simulink model "P4p2_integral"  (R2015a)
settings: Solver=ode1  StartTime=0.0  StopTime=inf  FixedStep=0.002  RelTol=1e-3
PostLoadFcn:
  | qc_set_target_type(getConfigSet(bdroot, 'QUARC Default Target Configuration'));
values from neighbouring files (symbols this model uses):
  A_hat = [0 1 0 0 0 0; zeros(1, 6); 0 0 0 1 0 0;zeros(1, 6); 0 0 0 0 0 1; k_3 0 0 0 0 0]    [P4p2_init.m]    (also in P4p3_init.m; p4p2_integral_init.m)
  B_hat = [0 0 ;0 k_1; 0 0; k_2 0; 0 0; 0 0]    [P4p2_init.m]    (also in P4p3_init.m; p4p2_integral_init.m)
  C_hat = [[1 0 0 0 0 0];[0 0 1 0 0 0]; [0 0 0 0 1 0]]    [P4p2_init.m]    (also in P4p3_init.m = [[0 0 1 0 0 0]; [0 0 0 0 1 0]]; p4p2_integral_init.m)
  K = lqr(A_reg, B_reg, Q_reg, R_reg)    [P4p2_init.m]    (also in P4p3_init.m; p4p2_integral_init.m)
  L = place(A_hat', C_hat', poles)'    [P4p2_init.m]    (also in P4p3_init.m; p4p2_integral_init.m)
  P = inv(C_reg*inv(B_reg*K-A_reg)*B_reg)    [P4p2_init.m]    (also in P4p3_init.m = inv(C*inv(B*K_new-A)*B); p4p2_integral_init.m = inv(C*inv(B*K_new-A)*B))
undefined symbols (not defined in the file or in its folder): HIL, Joystick_gain_x, Joystick_gain_y, qc_get_step_size, V_ss
libraries: simulink_extras x6, quarc_library x4
settings Model: SimulationMode=external  CovSFcnEnable=off  ExtModeTrigDuration=1000000  Creator=Rchan  LastModifiedBy=aashil
settings SolverCC: PositivePriorityOrder=on
settings DataIOCC: SignalLoggingSaveFormat=ModelDataLogs
settings OptimizationCC: ExpressionDepthLimit=2147483647  InitFltsAndDblsToZero=on
settings DebuggingCC: SaveWithParameterizedLinksMsg=none  UnderspecifiedInitializationDetection=Classic  MergeDetectMultiDrivingBlocksExec=none  SolverPrmCheckMsg=warning  MultiTaskDSMMsg=warning  MultiTaskCondExecSysMsg=none  FcnCallInpInsideContextMsg=UseLocalSettings  StateNameClashWarn=warning
settings RTWCC: SystemTargetFile=quarc_win64.tlc  TemplateMakefile=quarc_default_tmf  Description=QUARC Win64 Target
settings STFCustomTargetCC: TargetLibSuffix=.lib  TargetPreCompLibLocation=C:\PROGRA~3\QUARC\lib\2014a\win64\release  GenerateSampleERTMain=off  ConcurrentExecutionCompliant=on  GeneratePreprocessorConditionals=Disable all  ERTCustomFileBanners=off  SupportNonInlinedSFcns=on  SupportVariableSizeSignals=off  MATLABClassNameForMDSCustomization=Simulink.SoftwareTarget.GRTCustomization  CPPClassGenCompliant=on  GRTInterface=on  SystemTargetFile=quarc_win64.tlc
settings GRTTargetCC: TargetPreCompLibLocation=C:\PROGRA~3\QUARC\lib\2014a\win64\release  ParMdlRefBuildCompliant=off  CompOptLevelCompliant=off  CombineOutputUpdateFcns=off  MatFileLogging=off  GRTInterface=on  ExtMode=on  ExtModeMexFile=quarc_comm

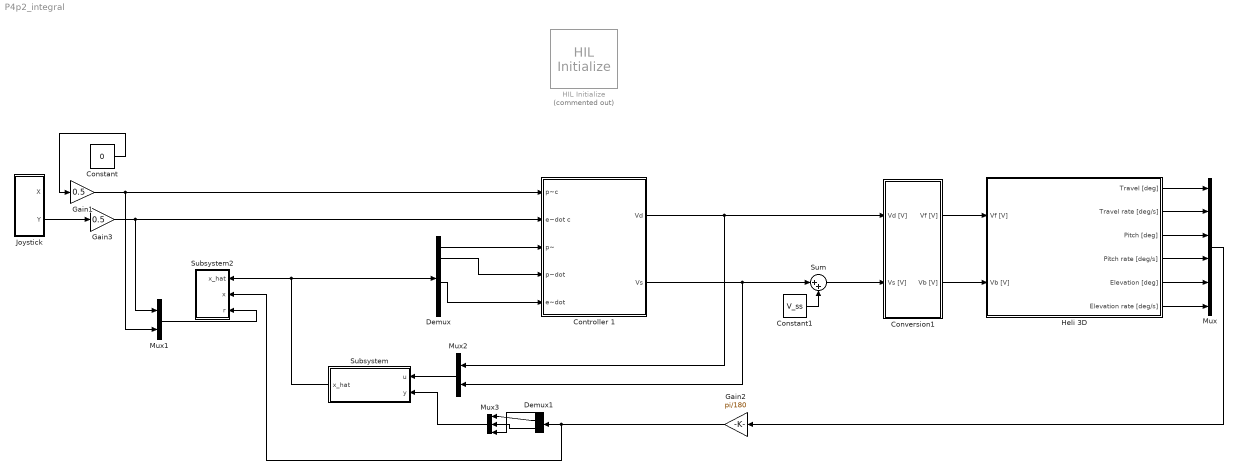
== system P4p2_integral ==
  Constant : Constant  Value=0
  Constant1 : Constant  Value=V_ss
  Controller 1 : Subsystem
  Conversion1 : Subsystem
  Demux : Demux  Outputs=6
  Demux1 : Demux  Outputs=6
  Gain1 : Gain  Gain=0.5
  Gain2 : Gain  Gain=pi/180
  Gain3 : Gain  Gain=0.5
  HIL Initialize : quarc_library/Data Acquisition/Generic/Configuration/HIL Initialize  Priority=-99  Commented=on  object_name=HIL-1  board_type=q8_usb  board_number=0  board_options=update_rate=normal;decimation=1  exclusive=off  active=off  hardware_clocks=[0:2]  clock_modes=[]  initial_clock_frequencies=[]  set_clock_params_at_start=off  set_clock_params_at_switch_in=off  set_clock_frequencies_at_start=off  set_clock_frequencies_at_switch_in=off  analog_input_channels=[0:7]  analog_input_maximums=10  analog_input_minimums=-10  set_analog_input_params_at_start=on  set_analog_input_params_at_switch_in=off  analog_output_channels=[0:7]  analog_output_maximums=10  analog_output_minimums=-10  initial_analog_outputs=[0]  final_analog_outputs=[0]  watchdog_analog_outputs=0  set_analog_output_params_at_start=on  set_analog_output_params_at_switch_in=off  set_analog_outputs_at_start=on  set_analog_outputs_at_switch_in=off  set_analog_outputs_at_terminate=on  set_analog_outputs_at_switch_out=off  set_analog_outputs_on_watchdog=off  digital_input_channels=[]  digital_output_channels=[]  digital_output_configuration=[]  initial_digital_outputs=[1]  final_digital_outputs=[1]  watchdog_digital_outputs=[1]  set_digital_output_params_at_start=off  set_digital_output_params_at_switch_in=off  set_digital_outputs_at_start=on  set_digital_outputs_at_switch_in=off  set_digital_outputs_at_terminate=on  set_digital_outputs_at_switch_out=off  set_digital_outputs_on_watchdog=off  encoder_channels=[0:7]  quadrature=[4]  encoder_filter_frequency=[]  initial_encoder_counts=[0]  set_encoder_params_at_start=on  set_encoder_params_at_switch_in=off  set_encoder_counts_at_start=on  set_encoder_counts_at_switch_in=off  pwm_channels=[0:7]  pwm_modes=0  pwm_frequency=99.532799999999995e6/4095  pwm_configuration=[0]  pwm_alignment=[0]  pwm_polarity=[1]  pwm_leading_deadband=[0]  pwm_trailing_deadband=[0]  initial_pwm_outputs=[0]  final_pwm_outputs=[0]  watchdog_pwm_outputs=[0]  set_pwm_params_at_start=on  set_pwm_params_at_switch_in=off  set_pwm_outputs_at_start=on  set_pwm_outputs_at_switch_in=off  set_pwm_outputs_at_terminate=on  set_pwm_outputs_at_switch_out=off  set_pwm_outputs_on_watchdog=off  other_output_channels=[]  initial_other_outputs=[]  final_other_outputs=[]  watchdog_other_outputs=[]  set_other_outputs_at_start=off  set_other_outputs_at_switch_in=off  set_other_outputs_at_terminate=off  set_other_outputs_at_switch_out=off  set_other_outputs_on_watchdog=off
  Heli 3D : Subsystem
  Joystick : Subsystem
  Mux : Mux  Inputs=6
  Mux1 : Mux  Inputs=2
  Mux2 : Mux  Inputs=2
  Mux3 : Mux  Inputs=3
  Subsystem : Subsystem
  Subsystem2 : Subsystem
  Sum : Sum  Inputs=|++
  wires:
  Conversion1/2(Vb [V]) -> Heli 3D/2(Vb [V])
  Conversion1/1(Vf [V]) -> Heli 3D/1(Vf [V])
  Heli 3D/1(Travel [deg]) -> Mux/1
  Heli 3D/2(Travel rate [deg/s]) -> Mux/2
  Heli 3D/3(Pitch [deg]) -> Mux/3
  Heli 3D/4(Pitch rate [deg/s]) -> Mux/4
  Heli 3D/5(Elevation [deg]) -> Mux/5
  Heli 3D/6(Elevation rate [deg/s]) -> Mux/6
  Mux/1 -> Gain2/1
  Joystick/2(Y) -> Gain3/1
  Gain3/1 -> Mux1/1, Controller 1/2(e~dot c)
  Constant/1 -> Gain1/1
  Mux1/1 -> Subsystem2/3(r)
  Gain1/1 -> Controller 1/1(p~c), Mux1/2
  Mux2/1 -> Subsystem/1(u)
  Subsystem/1(x_hat) -> Demux/1, Subsystem2/1(x_hat)
  Demux1/1 -> Mux3/3
  Demux1/3 -> Mux3/1
  Demux1/5 -> Mux3/2
  Mux3/1 -> Subsystem/2(y)
  Demux/1 -> Controller 1/3(p~)
  Demux/2 -> Controller 1/4(p~dot)
  Gain2/1 -> Subsystem2/2(x), Demux1/1
  Demux/4 -> Controller 1/5(e~dot)
  Controller 1/1("Vd ") -> Mux2/1, Conversion1/1(Vd [V])
  Constant1/1 -> Sum/2
  Sum/1 -> Conversion1/2(Vs [V])
  Controller 1/2(Vs) -> Sum/1, Mux2/2

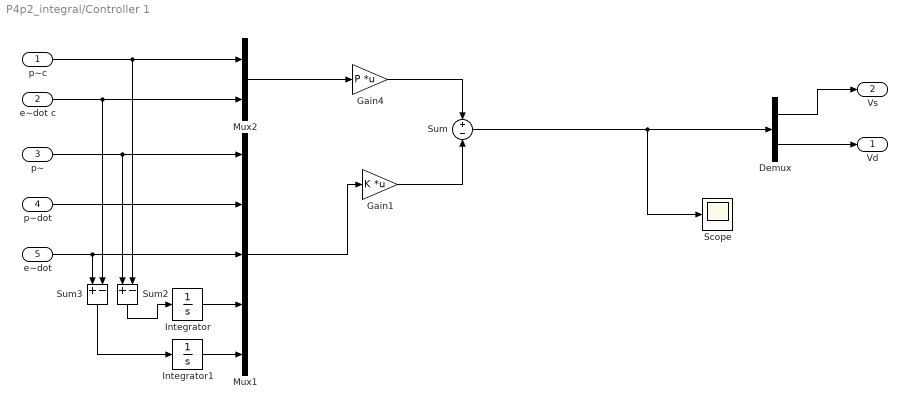
== system P4p2_integral/Controller 1 ==
  p~c : Inport
  e~dot c : Inport  Port=2
  p~ : Inport  Port=3
  p~dot : Inport  Port=4
  e~dot : Inport  Port=5
  Demux : Demux  Outputs=2
  Gain1 : Gain  Gain=K  Multiplication=Matrix(K*u)
  Gain4 : Gain  Gain=P  Multiplication=Matrix(K*u)
  Integrator : Integrator
  Integrator1 : Integrator
  Mux1 : Mux  Inputs=5
  Mux2 : Mux  Inputs=2
  Scope : Scope
      settings: YMin=-3.5  YMax=3
  Sum : Sum  Inputs=+-
  Sum2 : Sum  Inputs=+-
  Sum3 : Sum  Inputs=+-
  "Vd " : Outport
  Vs : Outport  Port=2
  wires:
  p~c/1 -> Mux2/1, Sum2/2
  p~dot/1 -> Mux1/2
  Gain1/1 -> Sum/2
  e~dot c/1 -> Mux2/2, Sum3/2
  Gain4/1 -> Sum/1
  Mux1/1 -> Gain1/1
  Sum/1 -> Scope/1, Demux/1
  Demux/2 -> "Vd "/1
  Mux2/1 -> Gain4/1
  Demux/1 -> Vs/1
  p~/1 -> Mux1/1, Sum2/1
  e~dot/1 -> Mux1/3, Sum3/1
  Integrator/1 -> Mux1/4
  Sum2/1 -> Integrator/1
  Integrator1/1 -> Mux1/5
  Sum3/1 -> Integrator1/1

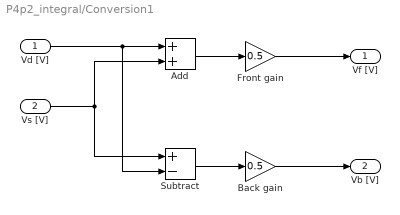
== system P4p2_integral/Conversion1 ==
  Vd [V] : Inport
  Vs [V] : Inport  Port=2
  Add : Sum
  Back gain : Gain  Gain=0.5
  Front gain : Gain  Gain=0.5
  Subtract : Sum  Inputs=+-
  Vf [V] : Outport
  Vb [V] : Outport  Port=2
  wires:
  Vd [V]/1 -> Subtract/2, Add/1
  Vs [V]/1 -> Subtract/1, Add/2
  Subtract/1 -> Back gain/1
  Back gain/1 -> Vb [V]/1
  Add/1 -> Front gain/1
  Front gain/1 -> Vf [V]/1

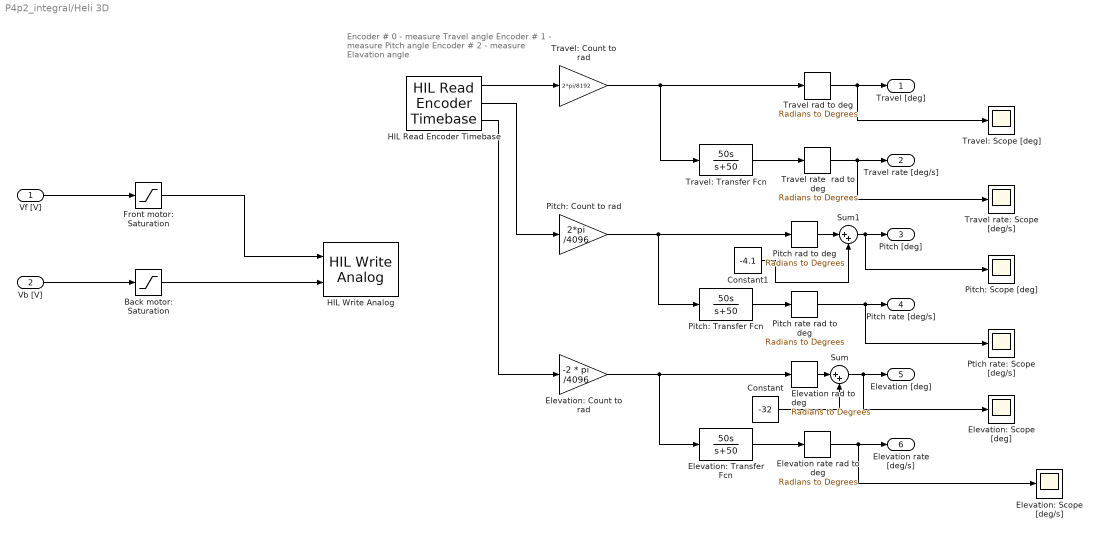
== system P4p2_integral/Heli 3D ==
  note: Encoder # 0 - measure Travel angle
      | Encoder # 1 - measure Pitch angle
      | Encoder # 2 - measure Elavation angle
  Vf [V] : Inport
  Vb [V] : Inport  Port=2
  Back motor: Saturation : Saturate  UpperLimit=5  LowerLimit=-5
  Constant : Constant  Value=-32
  Constant1 : Constant  Value=-4.1
  Elevation rad to deg : simulink_extras/Transformations/Radians to Degrees
  Elevation rate rad to deg : simulink_extras/Transformations/Radians to Degrees
  Elevation: Count to rad : Gain  Gain=-2 * pi /4096
  Elevation: Scope [deg/s] : Scope
      settings: YMin=-15  YMax=15  SaveName=ScopeData13
  Elevation: Scope [deg] : Scope
      settings: TimeRange=60  YMin=-32.5  YMax=15  SaveName=elevscope
  Elevation: Transfer Fcn : TransferFcn  Numerator=[50 0]  Denominator=[1 50]
  Front motor: Saturation : Saturate  UpperLimit=5  LowerLimit=-5
  HIL Read Encoder Timebase : quarc_library/Data Acquisition/Generic/Timebases/HIL Read Encoder Timebase  object_name=HIL-1  clock=0  channels=[0:2]  samples_in_buffer=max(ceil(1/qc_get_step_size), 1)  active=on  vector_output=off  data_type_mode=Inherit via back propagation  data_type=double
  HIL Write Analog : quarc_library/Data Acquisition/Generic/Immediate I//O/HIL Write Analog  object_name=HIL-1  channels=[0:1]  sample_time=-1  active=off  vector_input=off
  Pitch rad to deg : simulink_extras/Transformations/Radians to Degrees
  Pitch rate rad to deg : simulink_extras/Transformations/Radians to Degrees
  Pitch: Count to rad : Gain  Gain=2*pi /4096
  Pitch: Scope [deg] : Scope
      settings: TimeRange=600  YMin=-4  YMax=5.5  SaveName=pitchscope  MaxDataPoints=10000
  Pitch: Transfer Fcn : TransferFcn  Numerator=[50 0]  Denominator=[1 50]
  Ptich rate: Scope [deg/s] : Scope
      settings: TimeRange=600  YMin=-225  YMax=150  SaveName=pitchratescope
  Sum : Sum  Inputs=|++
  Sum1 : Sum  Inputs=|++
  Travel rad to deg : simulink_extras/Transformations/Radians to Degrees
  Travel rate  rad to deg : simulink_extras/Transformations/Radians to Degrees
  Travel rate: Scope [deg/s] : Scope
      settings: TimeRange=60  YMin=-55  YMax=30  SaveName=trratescope
  Travel: Count to rad : Gain  Gain=2*pi/8192
  Travel: Scope [deg] : Scope
      settings: TimeRange=60  YMin=-1750  YMax=250  SaveName=travelscope
  Travel: Transfer Fcn : TransferFcn  Numerator=[50 0]  Denominator=[1 50]
  Travel [deg] : Outport
  Travel rate [deg/s] : Outport  Port=2
  Pitch [deg] : Outport  Port=3
  Pitch rate [deg/s] : Outport  Port=4
  Elevation [deg] : Outport  Port=5
  Elevation rate [deg/s] : Outport  Port=6
  wires:
  HIL Read Encoder Timebase/1 -> Travel: Count to rad/1
  HIL Read Encoder Timebase/2 -> Pitch: Count to rad/1
  HIL Read Encoder Timebase/3 -> Elevation: Count to rad/1
  Travel: Count to rad/1 -> Travel: Transfer Fcn/1, Travel rad to deg/1
  Travel: Transfer Fcn/1 -> Travel rate  rad to deg/1
  Pitch: Count to rad/1 -> Pitch: Transfer Fcn/1, Pitch rad to deg/1
  Pitch: Transfer Fcn/1 -> Pitch rate rad to deg/1
  Elevation: Count to rad/1 -> Elevation: Transfer Fcn/1, Elevation rad to deg/1
  Elevation: Transfer Fcn/1 -> Elevation rate rad to deg/1
  Travel rad to deg/1 -> Travel: Scope [deg]/1, Travel [deg]/1
  Travel rate  rad to deg/1 -> Travel rate: Scope [deg/s]/1, Travel rate [deg/s]/1
  Pitch rate rad to deg/1 -> Ptich rate: Scope [deg/s]/1, Pitch rate [deg/s]/1
  Elevation rate rad to deg/1 -> Elevation: Scope [deg/s]/1, Elevation rate [deg/s]/1
  Vf [V]/1 -> Front motor: Saturation/1
  Vb [V]/1 -> Back motor: Saturation/1
  Front motor: Saturation/1 -> HIL Write Analog/1
  Back motor: Saturation/1 -> HIL Write Analog/2
  Sum/1 -> Elevation: Scope [deg]/1, Elevation [deg]/1
  Elevation rad to deg/1 -> Sum/1
  Constant/1 -> Sum/2
  Constant1/1 -> Sum1/2
  Pitch rad to deg/1 -> Sum1/1
  Sum1/1 -> Pitch: Scope [deg]/1, Pitch [deg]/1

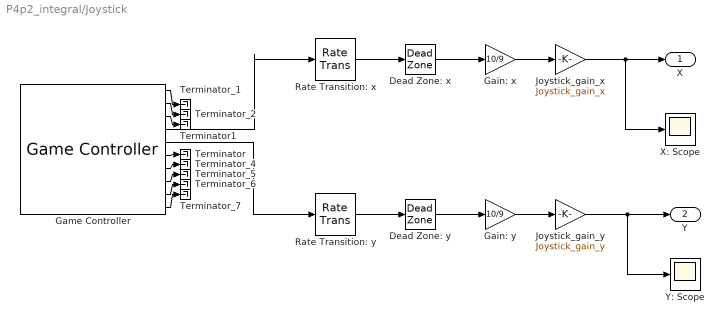
== system P4p2_integral/Joystick ==
  Dead Zone: x : DeadZone  LowerValue=-0.1  UpperValue=0.1  SaturateOnIntegerOverflow=on
  Dead Zone: y : DeadZone  LowerValue=-0.1  UpperValue=0.1  SaturateOnIntegerOverflow=on
  Gain: x : Gain  Gain=10/9
  Gain: y : Gain  Gain=10/9
  Game Controller : quarc_library/Devices/Peripherals/Target/Game Controller  controller=1  buffer_size=12  deadzone=[]  saturation=[]  sample_time=max(qc_get_step_size, 0.01)  auto_center=off  enabled=on
  Joystick_gain_x : Gain  Gain=Joystick_gain_x
  Joystick_gain_y : Gain  Gain=Joystick_gain_y
  Rate Transition: x : RateTransition
  Rate Transition: y : RateTransition
  Terminator : Terminator
  Terminator1 : Terminator
  Terminator_{1..2,4..7} (6 alike) : Terminator
  X: Scope : Scope
      settings: YMin=-1  YMax=1  SaveName=ScopeData7
  Y: Scope : Scope
      settings: YMin=-10  YMax=10  SaveName=ScopeData5
  X : Outport
  Y : Outport  Port=2
  wires:
  Rate Transition: y/1 -> Dead Zone: y/1
  Rate Transition: x/1 -> Dead Zone: x/1
  Game Controller/5 -> Rate Transition: y/1
  Game Controller/4 -> Rate Transition: x/1
  Game Controller/1 -> Terminator_1/1
  Game Controller/2 -> Terminator_2/1
  Game Controller/7 -> Terminator_4/1
  Game Controller/8 -> Terminator_5/1
  Game Controller/9 -> Terminator_6/1
  Game Controller/10 -> Terminator_7/1
  Game Controller/3 -> Terminator1/1
  Game Controller/6 -> Terminator/1
  Dead Zone: x/1 -> Gain: x/1
  Dead Zone: y/1 -> Gain: y/1
  Gain: x/1 -> Joystick_gain_x/1
  Gain: y/1 -> Joystick_gain_y/1
  Joystick_gain_x/1 -> X/1, X: Scope/1
  Joystick_gain_y/1 -> Y: Scope/1, Y/1

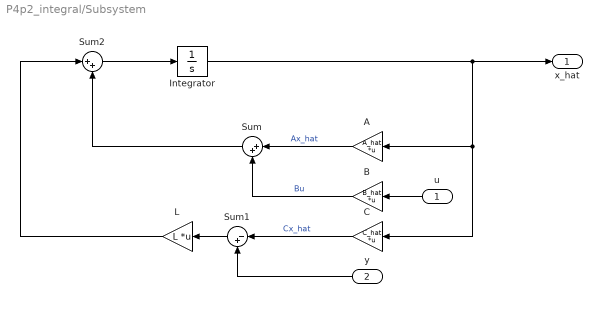
== system P4p2_integral/Subsystem ==
  u : Inport
  y : Inport  Port=2
  A : Gain  Gain=A_hat  Multiplication=Matrix(K*u)
  B : Gain  Gain=B_hat  Multiplication=Matrix(K*u)
  C : Gain  Gain=C_hat  Multiplication=Matrix(K*u)
  Integrator : Integrator
  L : Gain  Gain=L  Multiplication=Matrix(K*u)
  Sum : Sum  Inputs=|++
  Sum1 : Sum  Inputs=|-+
  Sum2 : Sum  Inputs=|++
  x_hat : Outport
  wires:
  u/1 -> B/1
  Sum2/1 -> Integrator/1
  A/1 -> Sum/1  "Ax_hat"
  B/1 -> Sum/2  "Bu"
  Integrator/1 -> C/1, A/1, x_hat/1
  C/1 -> Sum1/1  "Cx_hat"
  Sum1/1 -> L/1
  L/1 -> Sum2/1
  Sum/1 -> Sum2/2
  y/1 -> Sum1/2

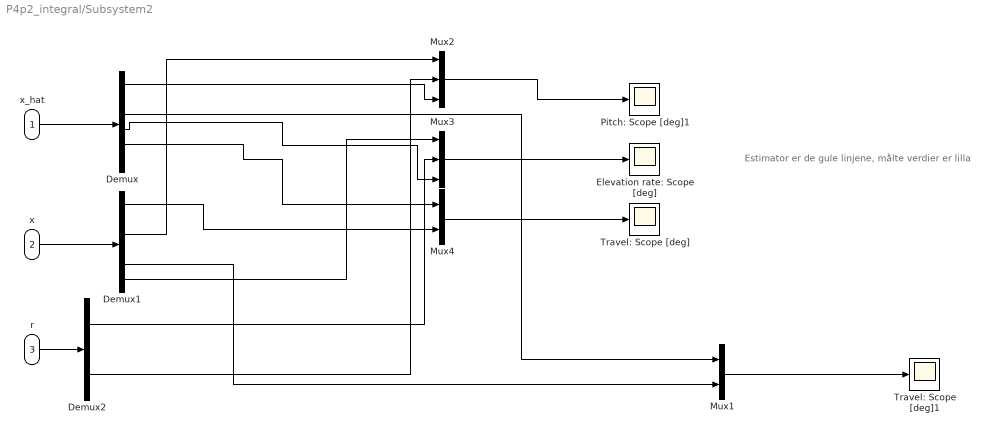
== system P4p2_integral/Subsystem2 ==
  note: Estimator er de gule linjene, målte verdier er lilla
  x_hat : Inport
  x : Inport  Port=2
  r : Inport  Port=3
  Demux : Demux  Outputs=6
  Demux1 : Demux  Outputs=6
  Demux2 : Demux  Outputs=2
  Elevation rate: Scope [deg] : Scope
      settings: TimeRange=60  YMin=-6.5  YMax=1  SaveName=elevation_hat
  Mux1 : Mux  Inputs=2
  Mux2 : Mux  Inputs=3
  Mux3 : Mux  Inputs=3
  Mux4 : Mux  Inputs=2
  Pitch: Scope [deg]1 : Scope
      settings: TimeRange=60  YMin=-0.9  YMax=0.8  SaveName=pitch_hat
  Travel: Scope [deg] : Scope
      settings: TimeRange=60  YMin=-7  YMax=3.5  SaveName=travel_hat
  Travel: Scope [deg]1 : Scope
      settings: TimeRange=60  YMin=-0.7  YMax=0.5  SaveName=travel_hat1
  wires:
  x/1 -> Demux1/1
  x_hat/1 -> Demux/1
  Mux4/1 -> Travel: Scope [deg]/1
  Mux3/1 -> Elevation rate: Scope [deg]/1
  Mux2/1 -> Pitch: Scope [deg]1/1
  Demux/1 -> Mux2/3
  Demux/4 -> Mux3/3
  Demux/5 -> Mux4/1
  Demux1/6 -> Mux3/1
  Demux1/1 -> Mux4/2
  Demux1/3 -> Mux2/1
  r/1 -> Demux2/1
  Demux2/1 -> Mux3/2
  Demux2/2 -> Mux2/2
  Mux1/1 -> Travel: Scope [deg]1/1
  Demux/3 -> Mux1/1
  Demux1/5 -> Mux1/2
